simulink model "L3_reg"  (Simulink 7.0)
settings: Solver=ode45  StartTime=0.0  StopTime=8  MaxStep=.01  RelTol=1e-7
values from neighbouring files (symbols this model uses):
  F = (C*(B*K-A)^-1 *B)^-1    [Systemregelung_ini.m]
  Fd = (s4d.c*(eye(size(A,1))-s4d.a+s4d.b*Kd)^-1 *s4d.b)^-1    [Systemregelung_ini.m]
  K = place(A,B,p)    [Systemregelung_ini.m]
  Kd = place(s4d.a,s4d.b,pd)    [Systemregelung_ini.m]
  T = .2    (= 0.2)    [Systemregelung_ini.m]
undefined symbols (not defined in the file or in its folder): A, B, C, D
Description:
  | SS-Model + SS-Controller
settings Model: Creator=Sz  LastModifiedBy=psz

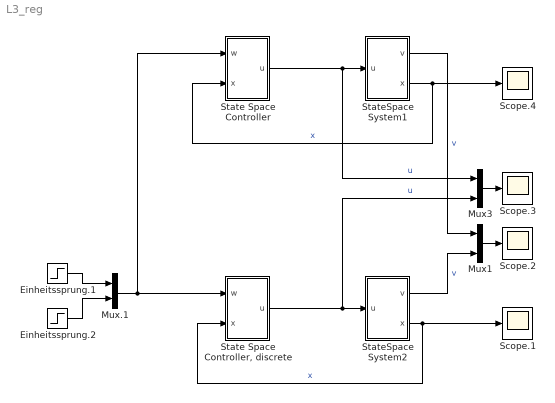
== system L3_reg ==
  Einheitssprung.1 : Step  Time=0  SampleTime=0
  Einheitssprung.2 : Step  Time=4  SampleTime=0
  Mux.1 : Mux  Inputs=2
  Mux1 : Mux  Inputs=2
  Mux3 : Mux  Inputs=2
  Scope.{1..4} (4 alike) : Scope
      Scope.1 settings: TimeRange=8  YMin=-0.5  YMax=4.5
      Scope.2 settings: TimeRange=8  YMin=-0.5  YMax=2.5
      Scope.3 settings: TimeRange=8  YMin=-3  YMax=6  SaveName=ScopeData2
      Scope.4 settings: TimeRange=8  YMin=-0.5  YMax=4.5  SaveName=ScopeData6
  State Space Controller : Subsystem  mask(State Space Controller){K=K, F=F}
  "State Space Controller, discrete" : Subsystem  mask(State Space Controller){KK=Kd, F=Fd, Ts=T}
      mask prompts: KK "K:"; Ts "Sample Time Ts:"
  StateSpace System1 : Subsystem  mask(State Space System){A=A, B=B, C=C, D=D}
  StateSpace System2 : Subsystem  mask(State Space System){A=A, B=B, C=C, D=D}
  wires:
  "State Space Controller, discrete"/1(u) -> StateSpace System2/1(u), Mux3/2  "u"
  StateSpace System2/2(x) -> Scope.1/1, "State Space Controller, discrete"/2(x)  "x"
  Einheitssprung.1/1 -> Mux.1/1
  Einheitssprung.2/1 -> Mux.1/2
  Mux.1/1 -> "State Space Controller, discrete"/1(w), State Space Controller/1(w)
  StateSpace System1/1(v) -> Mux1/1  "v"
  State Space Controller/1(u) -> StateSpace System1/1(u), Mux3/1  "u"
  StateSpace System1/2(x) -> Scope.4/1, State Space Controller/2(x)  "x"
  StateSpace System2/1(v) -> Mux1/2  "v"
  Mux1/1 -> Scope.2/1
  Mux3/1 -> Scope.3/1

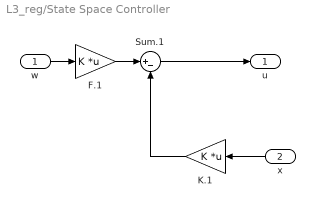
== system L3_reg/State Space Controller ==
  w : Inport
  x : Inport  Orientation=left  Port=2
  F.1 : Gain  Gain=K  Multiplication=Matrix(K*u)  ParameterDataType=sfix(16)  ParameterScaling=2^0  OutDataType=sfix(16)  OutScaling=2^0  SaturateOnIntegerOverflow=on  mask(P){K=F}
      mask prompts: K "F:"
      mask help: Proportionalelement
      mask Display: disp('F')
  K.1 : Gain  Orientation=left  Gain=K  Multiplication=Matrix(K*u)  ParameterDataType=sfix(16)  ParameterScaling=2^0  OutDataType=sfix(16)  OutScaling=2^0  SaturateOnIntegerOverflow=on  mask(P){K=K}
      mask help: Proportionalelement
      mask Display: disp('K')
  Sum.1 : Sum  Inputs=|+-  OutDataType=sfix(16)  OutScaling=2^0  SaturateOnIntegerOverflow=on  InputSameDT=on
  u : Outport
  wires:
  K.1/1 -> Sum.1/2
  F.1/1 -> Sum.1/1
  x/1 -> K.1/1
  Sum.1/1 -> u/1
  w/1 -> F.1/1

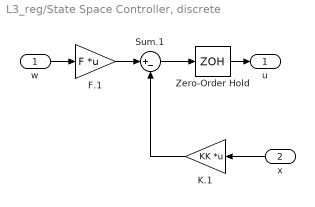
== system L3_reg/State Space Controller, discrete ==
  w : Inport
  x : Inport  Orientation=left  Port=2
  F.1 : Gain  Gain=F  Multiplication=Matrix(K*u)  ParameterDataType=sfix(16)  ParameterScaling=2^0  OutDataType=sfix(16)  OutScaling=2^0  SampleTime=Ts  SaturateOnIntegerOverflow=on  mask(P){F=F, Ts=-1}
      mask prompts: Ts "Sample Time Ts:"
      mask help: Proportionalelement
      mask Display: disp('F')
  K.1 : Gain  Orientation=left  Gain=KK  Multiplication=Matrix(K*u)  ParameterDataType=sfix(16)  ParameterScaling=2^0  OutDataType=sfix(16)  OutScaling=2^0  SaturateOnIntegerOverflow=on  mask(P){KK=KK, Ts=Ts}
      mask prompts: KK "K"; Ts "Sample Time Ts:"
      mask help: Proportionalelement
      mask Display: disp('K')
  Sum.1 : Sum  Inputs=|+-  OutDataType=sfix(16)  OutScaling=2^0  SaturateOnIntegerOverflow=on  InputSameDT=on
  Zero-Order Hold : ZeroOrderHold  SampleTime=Ts
  u : Outport
  wires:
  w/1 -> F.1/1
  Sum.1/1 -> Zero-Order Hold/1
  x/1 -> K.1/1
  F.1/1 -> Sum.1/1
  K.1/1 -> Sum.1/2
  Zero-Order Hold/1 -> u/1

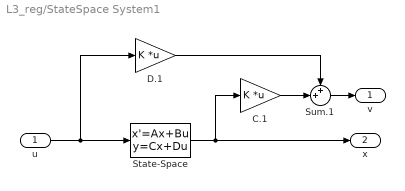
== system L3_reg/StateSpace System1 ==
  u : Inport
  C.1 : Gain  Gain=K  Multiplication=Matrix(K*u)  ParameterDataType=sfix(16)  ParameterScaling=2^0  OutDataType=sfix(16)  OutScaling=2^0  SaturateOnIntegerOverflow=on  mask(P){K=C}
      mask prompts: K "C:"
      mask help: Proportionalelement
      mask Display: disp('C')
  D.1 : Gain  Gain=K  Multiplication=Matrix(K*u)  ParameterDataType=sfix(16)  ParameterScaling=2^0  OutDataType=sfix(16)  OutScaling=2^0  SaturateOnIntegerOverflow=on  mask(P){K=D}
      mask prompts: K "D:"
      mask help: Proportionalelement
      mask Display: disp('D')
  State-Space : StateSpace  A=A  B=B  C=eye(size(A,1))  D=zeros(size(B))
  Sum.1 : Sum  Inputs=++|  OutDataType=sfix(16)  OutScaling=2^0  SaturateOnIntegerOverflow=on  InputSameDT=on
  v : Outport
  x : Outport  Port=2
  wires:
  State-Space/1 -> x/1, C.1/1
  u/1 -> State-Space/1, D.1/1
  C.1/1 -> Sum.1/2
  D.1/1 -> Sum.1/1
  Sum.1/1 -> v/1

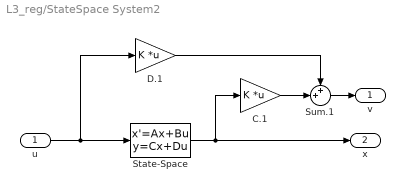
== system L3_reg/StateSpace System2 ==
  u : Inport
  C.1 : Gain  Gain=K  Multiplication=Matrix(K*u)  ParameterDataType=sfix(16)  ParameterScaling=2^0  OutDataType=sfix(16)  OutScaling=2^0  SaturateOnIntegerOverflow=on  mask(P){K=C}
      mask prompts: K "C:"
      mask help: Proportionalelement
      mask Display: disp('C')
  D.1 : Gain  Gain=K  Multiplication=Matrix(K*u)  ParameterDataType=sfix(16)  ParameterScaling=2^0  OutDataType=sfix(16)  OutScaling=2^0  SaturateOnIntegerOverflow=on  mask(P){K=D}
      mask prompts: K "D:"
      mask help: Proportionalelement
      mask Display: disp('D')
  State-Space : StateSpace  A=A  B=B  C=eye(size(A,1))  D=zeros(size(B))
  Sum.1 : Sum  Inputs=++|  OutDataType=sfix(16)  OutScaling=2^0  SaturateOnIntegerOverflow=on  InputSameDT=on
  v : Outport
  x : Outport  Port=2
  wires:
  State-Space/1 -> x/1, C.1/1
  u/1 -> State-Space/1, D.1/1
  C.1/1 -> Sum.1/2
  D.1/1 -> Sum.1/1
  Sum.1/1 -> v/1
